simulink model "bab"  (R2021a)
settings: Solver=VariableStepAuto  StartTime=0.0  StopTime=100  RelTol=1e-3
libraries: cstblocks x2, dspsrcs4 x1
settings Model: Creator=PC  LastModifiedBy=PC

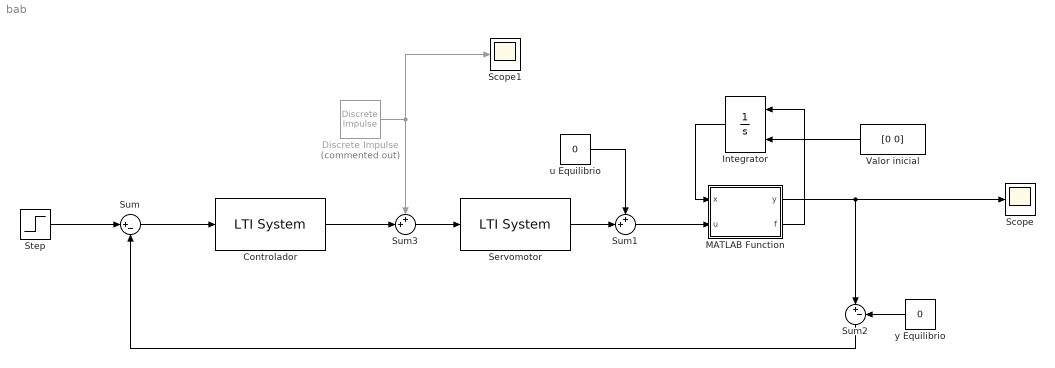
== system bab ==
  Controlador : cstblocks/LTI System  sys=Cdpd  IC=[]
  Discrete Impulse : dspsrcs4/Discrete  Impulse  Commented=on  Delay=0  SampleTime=1  FrameSample=1  OutputFrames=off  dataType=double  isSigned=on  wordLen=16  udDataType=sfix(16)  fracBitsMode=Best precision  numFracBits=15  OutDataTypeStr=double  LastOutDataTypeStr=double
  Integrator : Integrator  InitialConditionSource=external
  MATLAB Function : MATLAB Function  TreatAsAtomicUnit=on
  Scope : Scope
  Scope1 : Scope
  Servomotor : cstblocks/LTI System  sys=P_servo  IC=[]
  Step : Step  Time=0.1  After=0.25  SampleTime=0
  Sum : Sum  Inputs=|+-
  Sum1 : Sum  Inputs=++|
  Sum2 : Sum  Inputs=|+-
  Sum3 : Sum  Inputs=++|
  Valor inicial : Constant  Value=[0 0]
  u Equilibrio : Constant  Value=0
  y Equilibrio : Constant  Value=0
  wires:
  Step/1 -> Sum/1
  Sum/1 -> Controlador/1
  Sum1/1 -> MATLAB Function/2(u)
  u Equilibrio/1 -> Sum1/1
  MATLAB Function/1(y) -> Scope/1, Sum2/1
  y Equilibrio/1 -> Sum2/2
  Sum2/1 -> Sum/2
  MATLAB Function/2(f) -> Integrator/1
  Integrator/1 -> MATLAB Function/1(x)
  Valor inicial/1 -> Integrator/2
  Servomotor/1 -> Sum1/2
  Discrete Impulse/1 -> Sum3/1, Scope1/1
  Sum3/1 -> Servomotor/1
  Controlador/1 -> Sum3/2

== matlab function bab/MATLAB Function ==
  data: x input; u input; y output; f output
function [y, f] = fcn(x, u)
    
    g = 9.81;

    f1 = x(2);
    f2 = g*sin(u);

    y = x(1);
    f = [f1 f2];
end
